simulink model "ParallelSystem"  (R2014a)
settings: Solver=ode3  StartTime=0.0  StopTime=500  FixedStep=0.01  RelTol=1e-3
libraries: simulink x4
settings Model: SimulationMode=accelerator  Creator=nw010080  LastModifiedBy=nm010080
settings OptimizationCC: EfficientMapNaN2IntZero=off
settings DebuggingCC: UnderspecifiedInitializationDetection=Classic  StateNameClashWarn=warning
settings HardwareCC: TargetLongLongMode=on  TargetIntDivRoundTo=Zero  TargetEndianess=LittleEndian  TargetHWDeviceType=MATLAB Host  ProdEqTarget=off
settings CodeAppCC: MaxIdLength=128
settings GRTTargetCC: CombineOutputUpdateFcns=off  GRTInterface=on

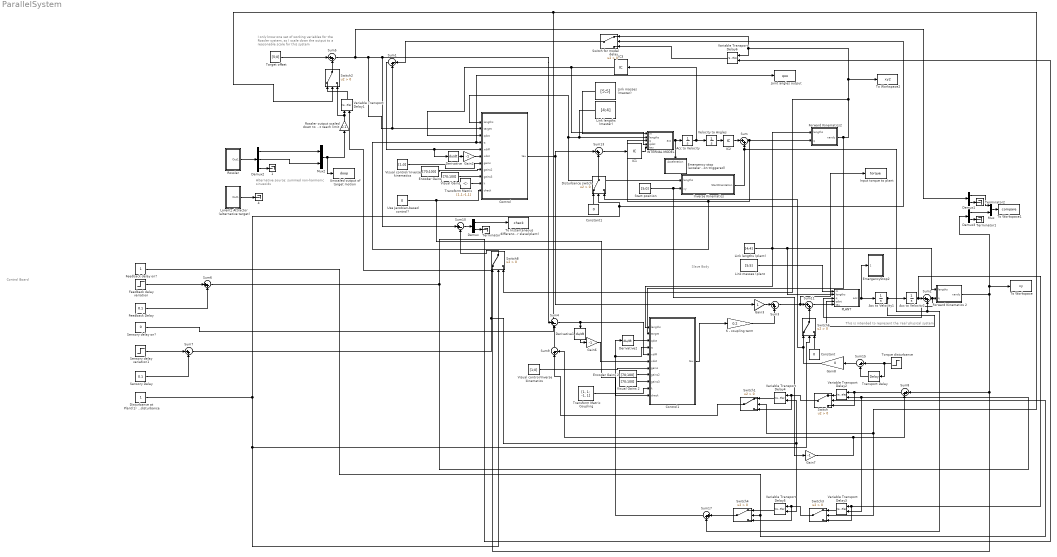
== system ParallelSystem ==
  note: Control Board
  note: Alternative source: summed
      | non-harmonic sinusoids
  note: Slave Body
  note: This is intended to represent the 'real' physical system
  note: I only know one set of working variables for
      | the Rossler system, so I scale down the output
      | to a reasonable scale for this system
  " 1" : Terminator
  " 4" : Terminator
  Acc to Velocity : Integrator
  Acc to Velocity1 : Integrator
  Acc to Velocity2 : Integrator
  Constant : Constant  Value=0
  Constant1 : Constant  Value=0
  Control : MATLAB Function  TreatAsAtomicUnit=on
  Control1 : MATLAB Function  TreatAsAtomicUnit=on
  Demux : Demux  Outputs=2
  Demux1 : Demux  Outputs=2
  Demux2 : Demux  Outputs=3
  Demux3 : Demux  Outputs=2
  Derivative : Derivative
  Derivative1 : Derivative
  Derivative2 : Derivative
  Disturbance switch : Switch  Criteria=u2 > Threshold
  "Disturbance at Plant(1) or Model(0)? (Setting to 0 also applies the feedback delay to the model, in order to observe the combined effect of delay and disturbance" : Constant
  Emergency stop (acceleration triggered) : Subsystem
  EmergencyStop2 : Subsystem
  Encoder Gains : Constant  Value=[70;100]
  Encoder Gains 2 : Constant  Value=[70;100]
  Feedback Delay : Constant  Value=0.1
  Feedback delay variation : Step  Time=200  After=0.06  SampleTime=0
  Feedback delay on? : Constant
  Forward Kinematics 2 : MATLAB Function  TreatAsAtomicUnit=on
  Forward Kinematics2 : MATLAB Function  TreatAsAtomicUnit=on
  Gain2 : Gain  Gain=-1
  Gain3 : Gain
  Gain6 : Gain  Gain=-1
  Gain7 : Gain  Gain=-1
  Gain8 : Gain  Gain=0
  IC1 : InitialCondition  Value=[0;0]
  IC2 : InitialCondition  Value=[0;0]
  IC3 : InitialCondition  Value=[0;0]
  INTERNAL MODEL : MATLAB Function  TreatAsAtomicUnit=on
  Input torque to plant : ToWorkspace  VariableName=torque  SaveFormat=Timeseries  SampleTime=-1
  Inverse Kinematics : MATLAB Function  TreatAsAtomicUnit=on
  Joint angles output : ToWorkspace  VariableName=qoo  SaveFormat=Timeseries  SampleTime=-1
  K - coupling term : Gain  Gain=0.2
  Link lengths (master) : Constant  Value=[4;4]
  Link lengths (plant) : Constant  Value=[4;4]
  Link masses (master) : Constant  Value=[5;5]
  Link masses (plant : Constant  Value=[5;5]
  Lorentz Attractor (alternative target) : Subsystem
  Mux : Mux  Inputs=2
  Mux2 : Mux  Inputs=2
  PLANT : MATLAB Function  TreatAsAtomicUnit=on
  Rossler : Subsystem
  Rossler output scaled down to accommodate robot reach limit : Gain  Gain=0.1
  Sensory Delay : Constant  Value=0.1
  Sensory delay variation1 : Step  Time=200  After=0.06  SampleTime=0
  Sensory delay on? : Constant  Value=0
  Start position : Constant  Value=[5;0]
  Sum{,2..3,5..8,11,13,17} (10 alike) : Sum  Inputs=|++
  Sum1 : Sum  Inputs=|-+
  Sum{4,9..10,15} (4 alike) : Sum  Inputs=|+-
  Switch{,1..4,6,8} (7 alike) : Switch  Criteria=u2 > Threshold
  Switch for model delay : Switch  Criteria=u2 > Threshold
  Target offset : Constant  Value=[5;0]
  Terminator : Terminator
  Terminator1 : Terminator
  Terminator2 : Terminator
  To Instantaneous difference between target and master or slave(plant) : ToWorkspace  VariableName=check  SaveFormat=Timeseries  SampleTime=-1
  To Workspace : ToWorkspace  VariableName=xy  SaveFormat=Timeseries  SampleTime=-1
  To Workspace1 : ToWorkspace  VariableName=compare  SaveFormat=Timeseries  SampleTime=-1
  To Workspace2 : ToWorkspace  VariableName=xy2  SaveFormat=Timeseries  SampleTime=-1
  Torque disturbance : Step  Time=200  SampleTime=0
  Transform Matrix : Constant  Value=[1,1;-1,1]
  Transform Matrix Coupling : Constant  Value=|
      | [1,    1;
      |    -1,    1]
  Transport Delay : TransportDelay  DelayTime=0.3
  Unscaled output of target motion : ToWorkspace  VariableName=doop  SaveFormat=Timeseries  SampleTime=-1
  Use Jacobian-based control? : Constant  Value=0
  Variable Transport Delay{1..5} (5 alike) : VariableTransportDelay  VariableDelayType=Variable transport delay  MaximumDelay=3  MaximumPoints=2048*2
  Variable Transport Delay6 : VariableTransportDelay  VariableDelayType=Variable transport delay  MaximumDelay=3  InitialOutput=[5;0]  MaximumPoints=2048*2
  Velocity to Angles : Integrator
  Visual Gains : Constant  Value=[70;100]
  Visual Gains 2 : Constant  Value=[70;100]
  Visual control/ Inverse kinematics : Constant  Value=[1;0]
  Visual control/Inverse kinematics : Constant  Value=[1;0]
  wires:
  INTERNAL MODEL/1(acc) -> Acc to Velocity/1, Emergency stop (acceleration triggered)/1(Acceleration)
  IC3/1 -> INTERNAL MODEL/4(qdot), Control/3(qdot)
  Encoder Gains/1 -> Control/8(gains2)
  PLANT/1(acc) -> EmergencyStop2/1(Acceleration), Acc to Velocity1/1
  Sum2/1 -> PLANT/3(q), Forward Kinematics 2/2(q)
  K - coupling term/1 -> Sum3/2
  Link masses (master)/1 -> INTERNAL MODEL/1(m)
  IC1/1 -> INTERNAL MODEL/5(tau)
  Link masses (plant/1 -> PLANT/1(m)
  Link lengths (plant)/1 -> Control1/1(lengths), Forward Kinematics2/1(lengths), PLANT/2(lengths), Forward Kinematics 2/1(lengths)
  Inverse Kinematics/1(StartOrientation) -> Sum/2, Sum17/2, Sum2/2
  Sum6/1 -> Variable Transport Delay6/2, Variable Transport Delay3/2, Variable Transport Delay2/2
  Visual Gains/1 -> Control/9(gains3)
  Transform Matrix/1 -> Control/10(k)
  Demux2/2 -> Mux2/2
  Demux2/1 -> Mux2/1
  Velocity to Angles/1 -> IC2/1
  IC2/1 -> Sum/1
  Gain3/1 -> Sum3/1
  Acc to Velocity/1 -> Velocity to Angles/1, IC3/1
  Derivative/1 -> Gain2/1
  Gain2/1 -> Control/6(xdot)
  Rossler output scaled down to accommodate robot reach limit/1 -> Switch2/3, Variable Transport Delay1/1
  Visual control/ Inverse kinematics/1 -> Control/7(gains)
  Mux2/1 -> Unscaled output of target motion/1, Rossler output scaled down to accommodate robot reach limit/1
  Demux2/3 -> " 1"/1
  Sum1/1 -> Derivative/1, Control/5(xdiff)
  Feedback Delay/1 -> Sum6/2
  Sensory Delay/1 -> Sum7/2
  Feedback delay variation/1 -> Sum6/1
  Sensory delay variation1/1 -> Sum7/1
  Sum8/1 -> Switch/3, Variable Transport Delay2/1
  Target offset/1 -> Sum5/1
  Lorentz Attractor (alternative target)/1(Out1) -> " 4"/1
  Rossler/1(Out1) -> Demux2/1
  Transform Matrix Coupling/1 -> Control1/10(k)
  Visual Gains 2/1 -> Control1/9(gains3)
  Gain6/1 -> Control1/6(xdot)
  Derivative1/1 -> Gain6/1
  Variable Transport Delay1/1 -> Switch2/1
  Sum11/1 -> PLANT/5(tau)
  Sum9/1 -> Sum4/2
  Sum4/1 -> Control1/5(xdiff), Derivative1/1
  Disturbance switch/1 -> Sum13/2
  Sum5/1 -> Demux1/1, Sum10/1, Sum4/1, Control/2(target), Sum1/2
  Sum15/1 -> Gain8/1
  Acc to Velocity1/1 -> Acc to Velocity2/1, PLANT/4(qdot)
  Control1/1(tau) -> K - coupling term/1
  Link lengths (master)/1 -> Control/1(lengths), Inverse Kinematics/1(lengths), INTERNAL MODEL/2(lengths)
  Variable Transport Delay2/1 -> Switch/1
  Variable Transport Delay4/1 -> Switch1/1
  Switch/1 -> Switch1/3, Variable Transport Delay4/1
  Switch2/1 -> Sum5/2
  Sensory delay on?/1 -> Switch2/2, Switch3/2, Switch1/2
  Feedback delay on?/1 -> Switch/2, Switch4/2
  Sum/1 -> Joint angles output/1, Control/4(q), INTERNAL MODEL/3(q), Forward Kinematics2/2(q)
  Torque disturbance/1 -> Transport Delay/1, Sum15/1
  Encoder Gains 2/1 -> Control1/8(gains2)
  Acc to Velocity2/1 -> Switch3/3, Variable Transport Delay3/1, Sum2/1
  Variable Transport Delay3/1 -> Switch3/1
  Variable Transport Delay5/1 -> Switch4/1
  Switch3/1 -> Variable Transport Delay5/1, Switch4/3
  Switch4/1 -> Sum17/1
  Visual control/Inverse kinematics/1 -> Control1/7(gains)
  Use Jacobian-based control?/1 -> Control1/11(check), Control/11(check)
  Derivative2/1 -> Control1/3(qdot)
  Switch1/1 -> Sum9/1
  Sum17/1 -> Control1/4(q), Derivative2/1
  Gain7/1 -> Sum9/2, Sum8/2
  Start position/1 -> Gain7/1, Inverse Kinematics/2(xy)
  Transport Delay/1 -> Sum15/2
  Forward Kinematics2/1(xandy) -> Control1/2(target), Switch8/3, Switch for model delay/1, Variable Transport Delay6/1, To Workspace2/1
  Sum10/1 -> Demux/1
  Demux/2 -> Terminator/1
  Demux/1 -> To Instantaneous difference between target and master or slave(plant)/1
  Switch6/1 -> Sum11/2
  Gain8/1 -> Disturbance switch/3, Switch6/1
  Constant/1 -> Switch6/3
  Constant1/1 -> Disturbance switch/1
  "Disturbance at Plant(1) or Model(0)? (Setting to 0 also applies the feedback delay to the model, in order to observe the combined effect of delay and disturbance"/1 -> Switch8/2, Switch6/2, Disturbance switch/2, Switch for model delay/2
  Variable Transport Delay6/1 -> Switch for model delay/3
  Sum7/1 -> Variable Transport Delay1/2, Variable Transport Delay4/2, Variable Transport Delay5/2
  Switch8/1 -> Sum10/2
  Mux/1 -> To Workspace1/1
  Demux1/1 -> Mux/1
  Demux3/1 -> Mux/2
  Demux3/2 -> Terminator1/1
  Demux1/2 -> Terminator2/1
  Forward Kinematics 2/1(xandy) -> Switch8/1, Sum8/1, To Workspace/1, Demux3/1
  Switch for model delay/1 -> Sum1/1
  Sum13/1 -> IC1/1
  Sum3/1 -> Input torque to plant/1, Sum11/1
  Control/1(tau) -> Sum13/1, Gain3/1

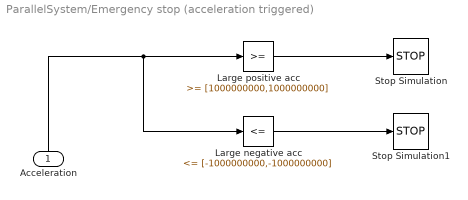
== system ParallelSystem/Emergency stop (acceleration triggered) ==
  Acceleration : Inport
  Large negative acc : simulink/Logic and Bit Operations/Compare To Constant  relop=<=  const=[-1000000000,-1000000000]  OutDataTypeStr=boolean
  Large positive acc : simulink/Logic and Bit Operations/Compare To Constant  relop=>=  const=[1000000000,1000000000]  OutDataTypeStr=boolean
  Stop Simulation : Stop
  Stop Simulation1 : Stop
  wires:
  Large negative acc/1 -> Stop Simulation1/1
  Large positive acc/1 -> Stop Simulation/1
  Acceleration/1 -> Large negative acc/1, Large positive acc/1

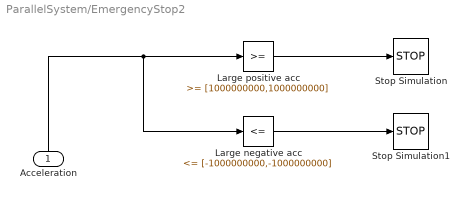
== system ParallelSystem/EmergencyStop2 ==
  Acceleration : Inport
  Large negative acc : simulink/Logic and Bit Operations/Compare To Constant  relop=<=  const=[-1000000000,-1000000000]  OutDataTypeStr=boolean
  Large positive acc : simulink/Logic and Bit Operations/Compare To Constant  relop=>=  const=[1000000000,1000000000]  OutDataTypeStr=boolean
  Stop Simulation : Stop
  Stop Simulation1 : Stop
  wires:
  Large negative acc/1 -> Stop Simulation1/1
  Large positive acc/1 -> Stop Simulation/1
  Acceleration/1 -> Large negative acc/1, Large positive acc/1

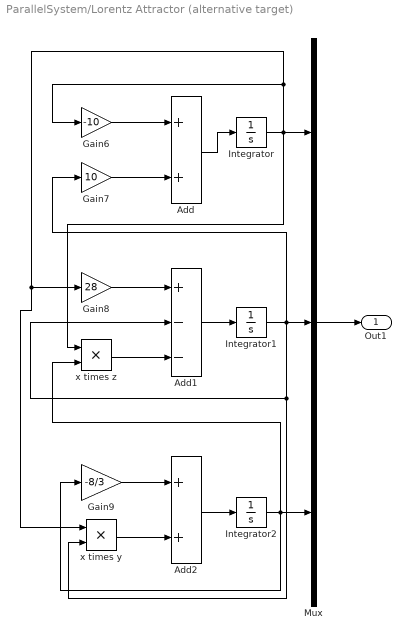
== system ParallelSystem/Lorentz Attractor (alternative target) ==
  Add : Sum
  Add1 : Sum  Inputs=+--
  Add2 : Sum
  Gain6 : Gain  Gain=-10
  Gain7 : Gain  Gain=10
  Gain8 : Gain  Gain=28
  Gain9 : Gain  Gain=-8/3
  Integrator : Integrator  InitialCondition=1
  Integrator1 : Integrator
  Integrator2 : Integrator
  Mux : Mux  Inputs=3
  x times y : Product
  x times z : Product
  Out1 : Outport
  wires:
  Add/1 -> Integrator/1
  Mux/1 -> Out1/1
  Gain7/1 -> Add/2
  Gain6/1 -> Add/1
  Integrator1/1 -> Mux/2, x times y/2, Add1/2, Gain7/1
  Add2/1 -> Integrator2/1
  Add1/1 -> Integrator1/1
  Integrator2/1 -> Mux/3, x times z/2, Gain9/1
  x times y/1 -> Add2/2
  Gain9/1 -> Add2/1
  x times z/1 -> Add1/3
  Integrator/1 -> Mux/1, x times z/1, x times y/1, Gain8/1, Gain6/1
  Gain8/1 -> Add1/1

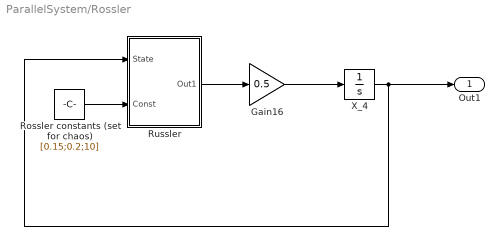
== system ParallelSystem/Rossler ==
  Gain16 : Gain  Gain=0.5
  Rossler constants (set for chaos) : Constant  Value=[0.15;0.2;10]
  Russler : Subsystem
  X_4 : Integrator  InitialCondition=[0;0;0]
  Out1 : Outport
  wires:
  X_4/1 -> Russler/1(State), Out1/1
  Gain16/1 -> X_4/1
  Russler/1(Out1) -> Gain16/1
  Rossler constants (set for chaos)/1 -> Russler/2(Const)

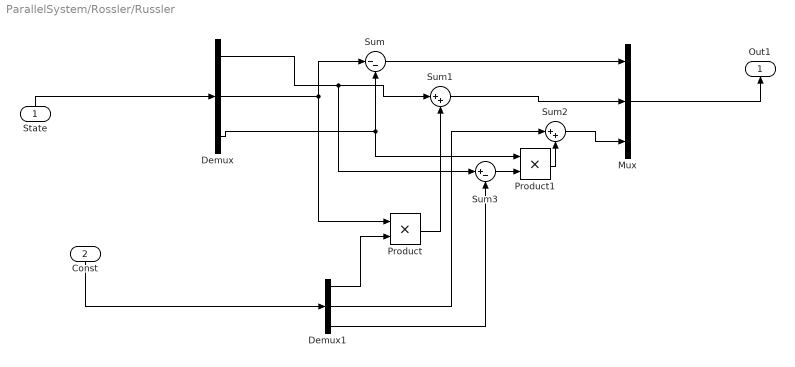
== system ParallelSystem/Rossler/Russler ==
  State : Inport
  Const : Inport  Port=2
  Demux : Demux  Outputs=3
  Demux1 : Demux  Outputs=3
  Mux : Mux  Inputs=3
  Product : Product
  Product1 : Product
  Sum : Sum  Inputs=|--
  Sum1 : Sum  Inputs=|++
  Sum2 : Sum  Inputs=|++
  Sum3 : Sum  Inputs=|+-
  Out1 : Outport
  wires:
  Demux1/2 -> Sum2/1
  Sum3/1 -> Product1/2
  Const/1 -> Demux1/1
  Demux/1 -> Sum3/1, Sum1/1
  Demux/2 -> Sum/1, Product/1
  Product1/1 -> Sum2/2
  Demux1/3 -> Sum3/2
  Sum/1 -> Mux/1
  Sum2/1 -> Mux/3
  Product/1 -> Sum1/2
  Mux/1 -> Out1/1
  Demux1/1 -> Product/2
  Sum1/1 -> Mux/2
  State/1 -> Demux/1
  Demux/3 -> Product1/1, Sum/2

== matlab function ParallelSystem/Forward Kinematics2 ==
  data: lengths input; xandy output; q input
function xandy  = fKinematics(lengths, q)
% find the position of the end effector using the arm forward kinematics
l1 = lengths(1);
l2 = lengths(2);

x = l1*cos(q(1)) + l2*cos(q(1)+q(2));
y = l1*sin(q(1)) + l2*sin(q(1)+q(2));

xandy = [x;y];

== matlab function ParallelSystem/Control ==
  data: lengths input; tau output; target input; qdot input; q input; xdiff input; xdot input; gains input; gains2 input; gains3 input; k input; check input
function tau  = control(lengths, target, qdot, q, xdiff, xdot, gains,gains2, gains3, k, check)
queue = q;% noise added to kinematic feedback
l1 = lengths(1);
l2 = lengths(2);

if(target(1)^2 + target(2)^2 > (l1+l2-0.02)^2)% caps target to within arm reach
    targ1 = target(1)*((l1+l2-0.02)/sqrt(target(1)^2+target(2)^2));
    targ2 = target(2)*((l1+l2-0.02)/sqrt(target(1)^2+target(2)^2));
    target = [targ1;targ2];
end


m1 = gains(1);
m2 = gains(2);
kp = gains3(1);
kv = gains3(2);
gp = gains2(1);
gv = gains2(2);


%approximate transform from workspace to jointspace
tau = [0;0];

M1 = [m1,0;0,m1];%camera gain
M2 = [m2,0;0,m2];%encoder gain

Kp = [kp,0;0,kp];% 'camera' position feedback gain
kv = [kv,0;0,kv];% 'camera' velocity feedback gain

Gp = [gp,0;0,gp];% jointspace position feedback gain
Gv = [gv,0;0,gv];% jointspace velocity feedback gain

%---------------------------------Inverse kinematics-----------------------
d1 = (target(1)^2 + target(2)^2 + l1^2 - l2^2)/(2*l1);
d2 = (target(1)^2 + target(2)^2 - l1^2 + l2^2)/(2*l2);

Q1 = atan2(target(2),target(1)) - atan2(sqrt(target(1)^2 + target(2)^2 - d1^2),d1);% error added to inverse kinematics
Q2 = atan2(sqrt(target(1)^2 + target(2)^2 - d1^2),d1) + atan2(sqrt(target(1)^2 + target(2)^2 - d2^2),d2);
%--------------------------------------------------------------------------

desiredq = [Q1;Q2];

J=[-l1*sin(q(1))-l2*sin(q(1)+q(2)), -l2*sin(q(1)+q(2)); l1*cos(q(1))+l2*cos(q(1)+q(2)), l2*cos(q(1)+q(2))];% Jacobian transpose
if(check)
    k = J';%J'/(J*J')
end

cam = M1*(Kp*k*(xdiff)-kv*k*xdot);% visual feedback terms
internal = M2*(Gp*(desiredq-queue)-Gv*qdot);%kinematic feedback terms

true = [-l1*sin(q(1))-l2*sin(q(1)+q(2)), -l2*sin(q(1)+q(2)); l1*cos(q(1))+l2*cos(q(1)+q(2)), l2*cos(q(1)+q(2))]'*xdot;
est = k*xdot;

angle = atan2(est(2),est(1))-atan2(true(2),true(1));% angle between true and estimated joint velocities

tau = cam + internal;% calculate total torque

== matlab function ParallelSystem/Inverse Kinematics ==
  data: lengths input; StartOrientation output; xy input
function StartOrientation  = iKinematics(lengths, xy)
% calculates the initial position of the arm using the arm inverse
% kinematics
l1 = lengths(1);
l2 = lengths(2);

StartOrientation = zeros(2,1);

d1 = (xy(1)^2 + xy(2)^2 + l1^2 - l2^2)/(2*l1);
d2 = (xy(1)^2 + xy(2)^2 - l1^2 + l2^2)/(2*l2);

StartOrientation(1) = atan2(xy(2),xy(1)) - atan2(sqrt(xy(1)^2 + xy(2)^2 - d1^2),d1);
StartOrientation(2) = atan2(sqrt(xy(1)^2 + xy(2)^2 - d1^2),d1) + atan2(sqrt(xy(1)^2 + xy(2)^2 - d2^2),d2);

== matlab function ParallelSystem/Control1 ==
  data: lengths input; tau output; target input; qdot input; q input; xdiff input; xdot input; gains input; gains2 input; gains3 input; k input; check input
function tau  = control(lengths, target, qdot, q, xdiff, xdot, gains,gains2, gains3, k,   check)
queue = q;% get joint angles
l1 = lengths(1);
l2 = lengths(2);

if(target(1)^2 + target(2)^2 > (l1+l2-0.02)^2)% caps target to within arm reach, ensuring inverse kinematics have real solutions
    targ1 = target(1)*((l1+l2-0.02)/sqrt(target(1)^2+target(2)^2));
    targ2 = target(2)*((l1+l2-0.02)/sqrt(target(1)^2+target(2)^2));
    target = [targ1;targ2];
end

% get gain values
m1 = gains(1);
m2 = gains(2);
kp = gains3(1);
kv = gains3(2);
gp = gains2(1);
gv = gains2(2);


% construct diagonal gain matrices
tau = [0;0];

M1 = [m1,0;0,m1];%camera gain
M2 = [m2,0;0,m2];%encoder gain

Kp = [kp,0;0,kp];% 'camera' position feedback gain
kv = [kv,0;0,kv];% 'camera' velocity feedback gain

Gp = [gp,0;0,gp];% jointspace position feedback gain
Gv = [gv,0;0,gv];% jointspace velocity feedback gain

%---------------------------------Inverse kinematics-----------------------
d1 = (target(1)^2 + target(2)^2 + l1^2 - l2^2)/(2*l1);
d2 = (target(1)^2 + target(2)^2 - l1^2 + l2^2)/(2*l2);

Q1 = atan2(target(2),target(1)) - atan2(sqrt(target(1)^2 + target(2)^2 - d1^2),d1);
Q2 = atan2(sqrt(target(1)^2 + target(2)^2 - d1^2),d1) + atan2(sqrt(target(1)^2 + target(2)^2 - d2^2),d2);
%--------------------------------------------------------------------------

desiredq = [Q1;Q2];

J=[-l1*sin(q(1))-l2*sin(q(1)+q(2)), -l2*sin(q(1)+q(2)); l1*cos(q(1))+l2*cos(q(1)+q(2)), l2*cos(q(1)+q(2))];% Jacobian transpose
if(check)
    k = J';% J'/(J*J')
end

cam = M1*(Kp*k*(xdiff)-kv*k*xdot);% visual feedback terms
internal = M2*(Gp*(desiredq-queue)-Gv*qdot);%kinematic feedback terms

% true = [-l1*sin(q(1))-l2*sin(q(1)+q(2)), -l2*sin(q(1)+q(2)); l1*cos(q(1))+l2*cos(q(1)+q(2)), l2*cos(q(1)+q(2))]'*xdot;
% est = k*xdot;
% 
% angle = atan2(est(2),est(1))-atan2(true(2),true(1));% angle between true and estimated joint velocities

tau = cam + internal;% calculate total torque

== matlab function ParallelSystem/INTERNAL MODEL ==
  data: m input; lengths input; acc output; q input; qdot input; tau input
function acc  = Dyn(m, lengths, q, qdot, tau)
queue = q;
acc = [0;0];

l1 = lengths(1);% length of link one
l2 = lengths(2);% length of link two
m1 = m(1);% mass of link one
m2 = m(2);% mass of link two

lc1 = l1/2;% distance to centre of mass of link one
lc2 = l2/2;% distance to centre of mass of link two

j1 = (m1*l1^2)/3;% moment of inertia for thin, ideal pole
j2 = (m2*l2^2)/3;

%%%%%%%%%%%%%%%%%%%%%%%%% inertia matrix %%%%%%%%%%%%%%%%%%%%%%%%%%%%%%%%%%
m11 = j1 + j2 +2*m2*l1*lc2*cos(queue(2)) + m2*l1^2 + m1*lc1^2 + m2*lc2^2;
m12 = j2 + m2*l1*lc2*cos(queue(2)) + m2*lc2^2;
m21 = m12;
m22 = j2 + m2*lc2^2;

M = [m11,m12;m21,m22];
%%%%%%%%%%%%%%%%%%%%%%%%%%%%%%%%%%%%%%%%%%%%%%%%%%%%%%%%%%%%%%%%%%%%%%%%%%%

%%%%%%%%%%%%%%%%%%%%%%%%%  coriolis force vector %%%%%%%%%%%%%%%%%%%%%%%%%%
h1 = -m2*l2*lc2*(2*qdot(1)+qdot(2))*qdot(2)*sin(queue(2));
h2 = m2*l1*lc2*qdot(1)^2*sin(queue(2));

h = [h1;h2];
%%%%%%%%%%%%%%%%%%%%%%%%%%%%%%%%%%%%%%%%%%%%%%%%%%%%%%%%%%%%%%%%%%%%%%%%%%%

acc = M\(tau-h);% solve dynamics equation for acceleration

== matlab function ParallelSystem/PLANT ==
  data: m input; lengths input; acc output; q input; qdot input; tau input
function acc  = Dyn(m, lengths, q, qdot, tau)
queue = q;
acc = [0;0];

l1 = lengths(1);% length of link one
l2 = lengths(2);% length of link two
m1 = m(1);% mass of link one
m2 = m(2);% mass of link two

lc1 = l1/2;% distance to centre of mass of link one
lc2 = l2/2;% distance to centre of mass of link two

j1 = (m1*l1^2)/3;% moment of inertia for thin, ideal pole
j2 = (m2*l2^2)/3;% placeholder

m11 = j1 + j2 +2*m2*l1*lc2*cos(queue(2)) + m2*l1^2 + m1*lc1^2 + m2*lc2^2;
m12 = j2 + m2*l1*lc2*cos(queue(2)) + m2*lc2^2;
m21 = m12;
m22 = j2 + m2*lc2^2;

M = [m11,m12;m21,m22];% inertia matrix


h1 = -m2*l2*lc2*(2*qdot(1)+qdot(2))*qdot(2)*sin(queue(2));% coriolis
h2 = m2*l1*lc2*qdot(1)^2*sin(queue(2));

h = [h1;h2];
acc = M\(tau-h);% solve dynamics equation for acceleration

== matlab function ParallelSystem/Forward Kinematics 2 ==
  data: lengths input; xandy output; q input
function xandy  = fKinematics(lengths, q)
% find the position of the end effector using the arm forward kinematics
l1 = lengths(1);
l2 = lengths(2);

x = l1*cos(q(1)) + l2*cos(q(1)+q(2));
y = l1*sin(q(1)) + l2*sin(q(1)+q(2));

xandy = [x;y];
